simulink model "exampleHeatTransfer2Ground"  (Simulink 7.6)
settings: Solver=ode45  StartTime=0.0  StopTime=365*24*3600  MaxStep=24*3600  RelTol=1e-3
libraries: carnot x1
settings Model: Creator=drhf  LastModifiedBy=drhf

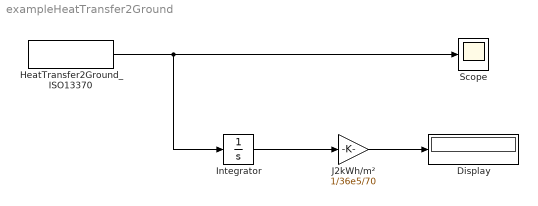
== system exampleHeatTransfer2Ground ==
  Display : Display
  HeatTransfer2Ground_ISO13370 : carnot/Load/Houses/heat_transfer/HeatTransfer2Ground_ISO13370  SystemSampleTime=-1  wallsize=[7 10]  gammat=0  Tmeaninside=23.8  deltathetai=3.8  Tmeanoutside=11  deltathetae=9.3  tshift=319*3600  dwall=0.4  cond_ground=2.0  cp_ground=800  rho_ground=2500  rtot=1./0.183
  Integrator : Integrator
  J2kWh/m² : Gain  Gain=1/36e5/70
  Scope : Scope
  wires:
  HeatTransfer2Ground_ISO13370/1 -> Scope/1, Integrator/1
  Integrator/1 -> J2kWh/m²/1
  J2kWh/m²/1 -> Display/1
